simulink model "hw2"  (R2013a)
settings: Solver=ode45  StartTime=0.0  StopTime=10.0  RelTol=1e-3
undefined symbols (not defined in the file): alpha, b, k, m, r
libraries: simulink x1
settings Model: Creator=admin  LastModifiedBy=admin

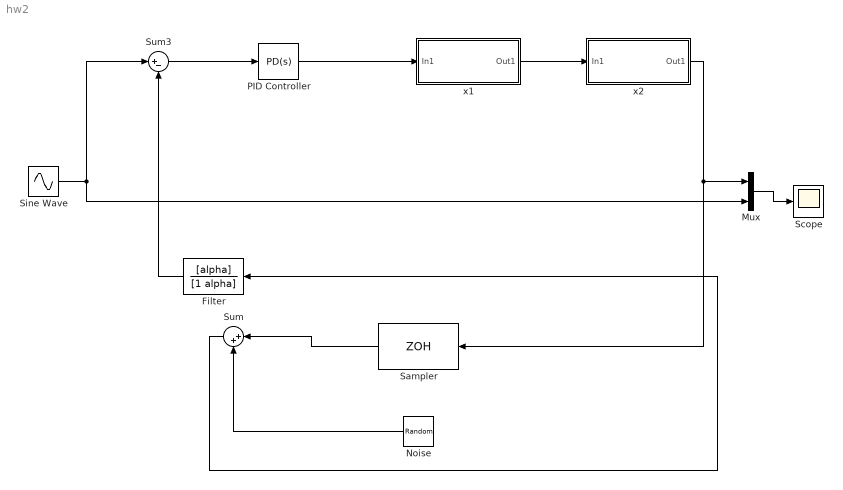
== system hw2 ==
  " Sampler " : ZeroOrderHold  SampleTime=0.005
  Filter : TransferFcn  Numerator=[alpha]  Denominator=[1 alpha]
  Mux : Mux  Inputs=2
  Noise : RandomNumber  Variance=0.01  SampleTime=0.005
  PID Controller : simulink/Continuous/PID Controller  Controller=PD  TimeDomain=Continuous-time  SampleTime=1  IntegratorMethod=Forward Euler  FilterMethod=Forward Euler  Form=Parallel  P=7.59237771354226  I=1  D=0.906683302383882  N=19.6860469438386  InitialConditionSource=internal  InitialConditionForIntegrator=0  InitialConditionForFilter=0  ExternalReset=none  LimitOutput=off  UpperSaturationLimit=inf  LowerSaturationLimit=-inf  LinearizeAsGain=on  AntiWindupMode=none  Kb=1  TrackingMode=off  Kt=1  PParamMin=[]  PParamMax=[]  IParamMin=[]  IParamMax=[]  DParamMin=[]  DParamMax=[]  NParamMin=[]  NParamMax=[]  KbParamMin=[]  KbParamMax=[]  KtParamMin=[]  KtParamMax=[]  POutMin=[]  POutMax=[]  IOutMin=[]  IOutMax=[]  DOutMin=[]  DOutMax=[]  NOutMin=[]  NOutMax=[]  KbOutMin=[]  KbOutMax=[]  KtOutMin=[]  KtOutMax=[]  IntegratorOutMin=[]  IntegratorOutMax=[]  FilterOutMin=[]  FilterOutMax=[]  SumOutMin=[]  SumOutMax=[]  SumI1OutMin=[]  SumI1OutMax=[]  SumI2OutMin=[]  SumI2OutMax=[]  SumI3OutMin=[]  SumI3OutMax=[]  SumDOutMin=[]  SumDOutMax=[]  SaturationOutMin=[]  SaturationOutMax=[]  IntegratorContinuousStateAttributes=''  IntegratorStateMustResolveToSignalObject=off  IntegratorRTWStateStorageClass=Auto  FilterContinuousStateAttributes=''  FilterStateMustResolveToSignalObject=off  FilterRTWStateStorageClass=Auto
  Scope : Scope
  Sine Wave : Sin  SampleTime=0
  Sum : Sum  Inputs=|++
  Sum3 : Sum  Inputs=|+-
  x1 : Subsystem
  x2 : Subsystem
  wires:
  Sine Wave/1 -> Mux/2, Sum3/1
  x2/1(Out1) -> " Sampler "/1, Mux/1
  x1/1(Out1) -> x2/1(In1)
  Sum3/1 -> PID Controller/1
  PID Controller/1 -> x1/1(In1)
  Mux/1 -> Scope/1
  " Sampler "/1 -> Sum/1
  Noise/1 -> Sum/2
  Filter/1 -> Sum3/2
  Sum/1 -> Filter/1

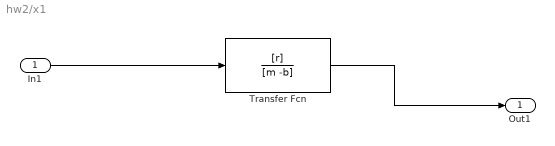
== system hw2/x1 ==
  In1 : Inport
  Transfer Fcn : TransferFcn  Numerator=[r]  Denominator=[m -b]
  Out1 : Outport
  wires:
  Transfer Fcn/1 -> Out1/1
  In1/1 -> Transfer Fcn/1

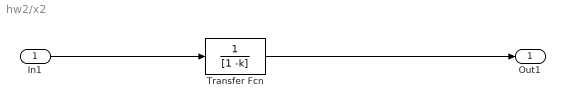
== system hw2/x2 ==
  In1 : Inport
  Transfer Fcn : TransferFcn  Denominator=[1 -k]
  Out1 : Outport
  wires:
  In1/1 -> Transfer Fcn/1
  Transfer Fcn/1 -> Out1/1
